simulink library "jMPClib"  (R2022b)
settings: Solver=ode45  StartTime=0.0  StopTime=10.0  RelTol=1e-3  EnableMultiTasking=on
undefined symbols (not defined in the file or in its folder): iter, lam0, MPC1, Plant, sigma, t0, titles, tlim, tol, vrw, ylims, z0
libraries: simulink x2, dspindex x2, $bdroot x1
settings Model: Creator=jocurrie  LastModifiedBy=Jonathan Currie
settings SolverCC: AlgebraicLoopSolver=TrustRegion
settings DataIOCC: LimitDataPoints=on  SaveFormat=Array  SignalLoggingSaveFormat=ModelDataLogs  ReturnWorkspaceOutputs=off
settings OptimizationCC: ExpressionDepthLimit=2147483647  LifeSpan=inf
settings DebuggingCC: UnderspecifiedInitializationDetection=Classic  MergeDetectMultiDrivingBlocksExec=none  SolverPrmCheckMsg=warning  FcnCallInpInsideContextMsg=warning  UnconnectedInputMsg=warning  UnconnectedOutputMsg=warning  UnconnectedLineMsg=warning  StateNameClashWarn=warning  SFUnexpectedBacktrackingDiag=warning  SFNoUnconditionalDefaultTransitionDiag=warning  SFExecutionAtInitializationDiag=none  SFMachineParentedDataDiag=warning  ArithmeticOperatorsInVariantConditions=warning
settings HardwareCC: ProdBitPerPointer=32  ProdBitPerSizeT=32  ProdBitPerPtrDiffT=32  ProdLargestAtomicFloat=None  ProdIntDivRoundTo=Undefined  ProdEndianess=Unspecified  ProdWordSize=32  ProdHWDeviceType=32-bit Generic
settings ModelReferenceCC: PropagateSignalLabelsOutOfModel=off
settings SFSimCC: SimUseLocalCustomCode=off  CustomCodeUndefinedFunction=UseInterfaceOnly
settings RTWCC: RTWUseLocalCustomCode=off
settings CodeAppCC: StateflowObjectComments=on
settings GRTTargetCC: TargetLangStandard=C89/C90 (ANSI)  CombineOutputUpdateFcns=off  GRTInterface=on
settings ConfigComp: CovMetricSettings=dw  CovSaveCumulativeToWorkspaceVar=on  CovSaveSingleToWorkspaceVar=on  CovExternalEMLEnable=off

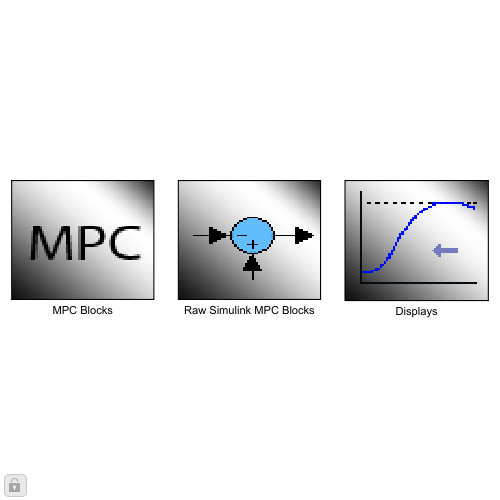
[thumbnail: Simulink's stored preview of the top-level diagram]
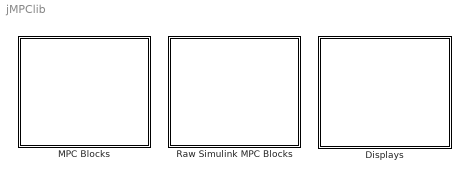
== system jMPClib ==
  Displays : Subsystem
      mask Display: image(imread('Images/scrollplot.png'))
  MPC Blocks : Subsystem
      mask Display: image(imread('Images/mpcblock.png'))
  Raw Simulink MPC Blocks : Subsystem
      mask Display: image(imread('Images/rawsim.png'))

== system jMPClib/Displays ==
  3D Simulation with Scopes : M-S-Function  FunctionName=sfun_3Dwgraph  Parameters=vrw,titles,ylims,tlim,viden  mask(jMPC 3D Simulation Interface){vrw=vrw, titles=titles, limits=ylims, tlim=tlim, viden=0}
      mask prompts: vrw "VR World"; titles "Scope Titles (Cell Array)"; limits "Scope Y Limits (Cell Array)"; tlim "Scope T Limit"; viden "Enable Video Output"
      mask help:
      | Allows the Simulink 3D interface to be run with live scrolling scopes showing runtime data.
      |
      | VR World - The VRML 3D World file name
      | Titles   - A cell array of titles to appear above each scope
      | Y Limits - A cell array of the y axis limits of each scope
      | T Limit  - The length of time before all scopes begin to scroll
      | Video Out - Enable a video output of RGB matrices. Noticeably slows down simulation!
      settings: DestroyFcn=|
      | block = get_param(gcbh, 'Parent');
      | FigHandle = get_param(block, 'UserData');
      | if ~isempty(FigHandle)
      |   close(FigHandle);
      | end
      mask Display: image(imread('Images/3Dsim.png'));
  Scrolling Display : M-S-Function  FunctionName=sfun_scroll  Parameters=Ts,Frame_Size,Update_Delay,y_lim,setp  mask(Scrolling Plot){Ts=0.1, Frame_Size=200, Update_Delay=0.005, y_lim=[-1 1], setp=on}
      mask prompts: Ts "Sampling Time (Seconds)"; Frame_Size "Frame Size (Samples)"; Update_Delay "Update Delay (Seconds)"; y_lim "Initial Y axis Limits [ymin ymax]"; setp "Enable Set Point Input"
      mask help:
      | Create a scrolling, autoscaling display for use in Simulink
      |
      | The display is a discrete component, and requires a sampling period. Adjust this period for the desired resolution.
      |
      | Frame size refers to the number of samples to be displayed on the screen before it begins to scroll.
      |
      | Note this block accepts a maximum of one input per port, if you connect a multiple dimsension signal results will be unpredictable.
      |
      | Update delay allows a rough delay of the simulation execution period, allowing the user to slow down the display.
      mask init:
      | if(~Ts)
      |     disp('Warning: Sampling Time (Ts) Not Specifed or is Zero');
      |     Ts = 0.1;
      | end
      | 
      | if(~Frame_Size)
      |     disp('Warning: Frame Size Not Specifed or is Zero');
      |     Frame_Size = 100;
      | end
      | 
      | if(Update_Delay < 0)
      |     Update_Delay = 0;
      | else if(Update_Delay > 10)
      |         disp('Warning: Update Delay Specified as > 10'); 
      |         Update_Delay = 10;
      |     end
      | end
      | 
      | if(y_lim(1) > y_lim(2))
      |     disp('Warning: Limit 1 is greater than Limit 2');
      |     y_lim(1) = -y_lim(1);
      | end
      | if(y_lim(1) == y_lim(2))
      |     disp('Warning: Limits are equal');
      |     if(~y_lim(1))
      |         y_lim(2) = 1;
      |     else
      |         y_lim(2) = y_lim(2)+abs(y_lim(2));
      |     end
      | end
      mask Help: web('jMPC_Simulink_scroll.html', '-helpbrowser');
      mask Display: image(imread('Images/Scrollpic.jpg'))

== system jMPClib/MPC Blocks ==
  Continuous ODE Plant : M-S-Function  FunctionName=sfun_jNL  Parameters=jNLObj  mask(Continuous ODE Model){jNLObj=Plant}
      mask prompts: jNLObj "jNL Object"
      mask help:
      | Implements a jNL object containing a function handle to an Ordinary Differential Equation (ODE) containing the state update equation.
      |
      | Accepts a jNL class object containing the model ODE function.
      mask Display:
      | image(imread('ode_plant.png'))
      | text(0.3,0.35,'dx/dt = f(x,u)')
      | port_label('output',1,'y ')
      | port_label('output',2,'x ')
      | port_label('input',1,' u')
  Discrete LTI Plant : Subsystem  mask(Discrete Linear Model){jSSobj=Plant}
      mask prompts: jSSobj "jSS Object"
      mask help:
      | x(k+1)  = Ax(k) + Bu(k)
      | y(k+1)  = Cx(k+1)
      |
      | Accepts a jSS class object containing the model SS matrices.
      mask Help: web('jMPC_Simulink_displant.html', '-helpbrowser');
      mask Display:
      | image(imread('Images/ltiplant.png'))
      | text(0.3,0.35,'x+1 = Ax+Bu')
      | port_label('output',1,'y ')
      | port_label('output',2,'x ')
      | port_label('input',1,' u')
  Discrete MPC Controller : Subsystem  mask(Model Predictive Controller){SIMJMPC=MPC1}
      mask prompts: SIMJMPC "jMPC Object"
      mask help:
      | MPC implemented as a C-MEX S Function for accelerated MPC simulations.
      |
      | Accepts a jMPC class object containing the controller specification.
      mask Help: web('jMPC_Simulink_dismpcs.html', '-helpbrowser');
      mask Display:
      | image(imread('Images/MPCPic.png'));
      | port_label('input',1,'mdist');
      | port_label('input',2,'setp');
      | port_label('input',3,'yp');
      | port_label('output',1,'u');
      | port_label('output',2,'delu');
      | port_label('output',4,'xm');
      | port_label('output',3,'ym');
      | port_label('output',5,'stats');

== system jMPClib/Raw Simulink MPC Blocks ==
  Discrete MPC (Raw Simulink) : Subsystem  mask(Model Predictive Controller){J=MPC1}
      mask prompts: J "jMPC Object"
      mask help:
      | General MPC for simulation (states and model output viewable).
      |
      | Accepts a jMPC class object containing the controller specification.
      mask Help: web('jMPC_Simulink_dismpc.html', '-helpbrowser');
      mask Display:
      | image(imread('Images/MPCPic2.png'));
      | port_label('input',1,'setp');
      | port_label('input',2,'yp');
      | port_label('output',1,'u');
      | port_label('output',2,'delu');
      | port_label('output',4,'xm');
      | port_label('output',3,'ym');
  Wright QP Solver : Subsystem  mask(Quadratic Programming Solver){iter=iter, tol=tol, z0=z0, lam0=lam0, t0=t0, esig=sigma}
      mask prompts: iter "Maximum Iterations"; tol "Solver Tolerance"; z0 "Initial z (ndec x 1)"; lam0 "Initial lambda (ncon x 1)"; t0 "Initial t (ncon x 1)"; esig "Sigma Array (ncon x 1)"
      mask help: QP Solver for MPC using Wright's Method
      mask Help: web('jMPC_Simulink_wright.html', '-helpbrowser');
      mask Display:
      | image(imread('Images/WrightPic.jpg'));
      | port_label('input',1,'H');
      | port_label('input',2,'f');
      | port_label('input',3,'A');
      | port_label('input',4,'b');
      | port_label('output',1,'Solution');
      | port_label('output',2,'Iterations');

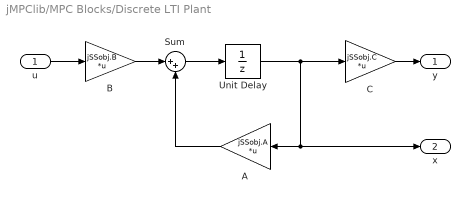
== system jMPClib/MPC Blocks/Discrete LTI Plant ==
  u : Inport
  A : Gain  Gain=jSSobj.A  Multiplication=Matrix(K*u)
  B : Gain  Gain=jSSobj.B  Multiplication=Matrix(K*u)
  C : Gain  Gain=jSSobj.C  Multiplication=Matrix(K*u)
  Sum : Sum  Inputs=|++
  Unit Delay : UnitDelay  InitialCondition=jSSobj.x0  SampleTime=-1  HasFrameUpgradeWarning=on
  y : Outport
  x : Outport  Port=2
  wires:
  C/1 -> y/1
  u/1 -> B/1
  Sum/1 -> Unit Delay/1
  B/1 -> Sum/1
  A/1 -> Sum/2
  Unit Delay/1 -> x/1, A/1, C/1

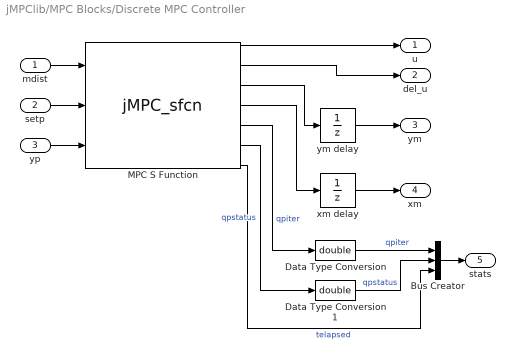
== system jMPClib/MPC Blocks/Discrete MPC Controller ==
  mdist : Inport
  setp : Inport  Port=2
  yp : Inport  Port=3
  Bus Creator : BusCreator  Inputs=3
  Data Type Conversion : DataTypeConversion  OutDataTypeStr=double  SaturateOnIntegerOverflow=off  RndMeth=Floor
  Data Type Conversion1 : DataTypeConversion  OutDataTypeStr=double  SaturateOnIntegerOverflow=off  RndMeth=Floor
  MPC S Function : S-Function  FunctionName=jMPC_sfcn  Parameters=SIMJMPC.Model.A,SIMJMPC.Model.B,SIMJMPC.Model.Ts,SIMJMPC.Np,SIMJMPC.Nb,SIMJMPC.pred,SIMJMPC.sizes,SIMJMPC.state_est,SIMJMPC.QP,SIMJMPC.index,SIMJMPC.constraints,SIMJMPC.initial,SIMJMPC.mpcopts,SIMJMPC.lin  SFunctionDeploymentMode=off  EnableBusSupport=off
  xm delay : UnitDelay  InitialCondition=SIMJMPC.initial.xm+SIMJMPC.lin.x_op  SampleTime=-1  HasFrameUpgradeWarning=on
  ym delay : UnitDelay  InitialCondition=SIMJMPC.initial.ym+SIMJMPC.lin.y_op_full  SampleTime=-1  HasFrameUpgradeWarning=on
  u : Outport
  del_u : Outport  Port=2
  ym : Outport  Port=3
  xm : Outport  Port=4
  stats : Outport  Port=5
  wires:
  MPC S Function/7 -> Bus Creator/3  "telapsed"
  Bus Creator/1 -> stats/1
  MPC S Function/3 -> ym delay/1
  MPC S Function/4 -> xm delay/1
  MPC S Function/1 -> u/1
  MPC S Function/2 -> del_u/1
  ym delay/1 -> ym/1
  xm delay/1 -> xm/1
  mdist/1 -> MPC S Function/1
  setp/1 -> MPC S Function/2
  yp/1 -> MPC S Function/3
  Data Type Conversion1/1 -> Bus Creator/2  "qpstatus"
  Data Type Conversion/1 -> Bus Creator/1  "qpiter"
  MPC S Function/5 -> Data Type Conversion/1  "qpiter"
  MPC S Function/6 -> Data Type Conversion1/1  "qpstatus"

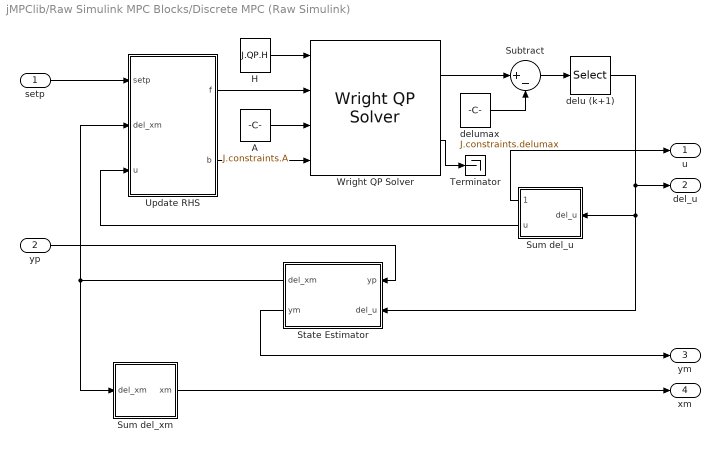
== system jMPClib/Raw Simulink MPC Blocks/Discrete MPC (Raw Simulink) ==
  setp : Inport
  yp : Inport  Port=2
  A : Constant  Value=J.constraints.A
  H : Constant  Value=J.QP.H
  State Estimator : Subsystem
  Subtract : Sum  Inputs=|+-
  Sum del_u : Subsystem
  Sum del_xm : Subsystem
  Terminator : Terminator
  Update RHS : Subsystem
  Wright QP Solver : $bdroot/Raw Simulink MPC Blocks/Wright QP Solver  iter=200  tol=1e-6  z0=J.QP.z0  lam0=J.QP.lam0  t0=J.QP.t0  esig=J.QP.sigma
  delu (k+1) : Selector  InputPortWidth=J.sizes.Nb_in  IndexOptions=Index vector (dialog)  Indices=1:J.sizes.n_in  OutputSizes=1
  delumax : Constant  Value=J.constraints.delumax
  u : Outport
  del_u : Outport  Port=2
  ym : Outport  Port=3
  xm : Outport  Port=4
  wires:
  H/1 -> Wright QP Solver/1
  A/1 -> Wright QP Solver/3
  Update RHS/1(f) -> Wright QP Solver/2
  Update RHS/2(b) -> Wright QP Solver/4
  Wright QP Solver/2 -> Terminator/1
  Wright QP Solver/1 -> Subtract/1
  Subtract/1 -> delu (k+1)/1
  delu (k+1)/1 -> del_u/1, State Estimator/2(del_u), Sum del_u/1(del_u)
  setp/1 -> Update RHS/1(setp)
  delumax/1 -> Subtract/2
  State Estimator/1(del_xm) -> Update RHS/2(del_xm), Sum del_xm/1(del_xm)
  yp/1 -> State Estimator/1(yp)
  Sum del_xm/1(xm) -> xm/1
  State Estimator/2(ym) -> ym/1
  Sum del_u/1(u (k+1)) -> u/1
  Sum del_u/2(u) -> Update RHS/3(u)

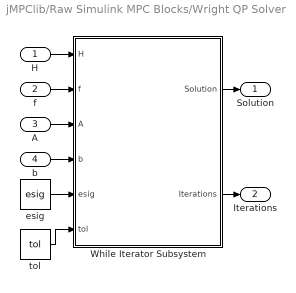
== system jMPClib/Raw Simulink MPC Blocks/Wright QP Solver ==
  H : Inport
  f : Inport  Port=2
  A : Inport  Port=3
  b : Inport  Port=4
  While Iterator Subsystem : Subsystem  TreatAsAtomicUnit=on
  esig : Constant  Value=esig
  tol : Constant  Value=tol
  Solution : Outport
  Iterations : Outport  Port=2
  wires:
  While Iterator Subsystem/2(Iterations) -> Iterations/1
  While Iterator Subsystem/1(Solution) -> Solution/1
  tol/1 -> While Iterator Subsystem/6(tol)
  esig/1 -> While Iterator Subsystem/5(esig)
  b/1 -> While Iterator Subsystem/4(b)
  A/1 -> While Iterator Subsystem/3(A)
  H/1 -> While Iterator Subsystem/1(H)
  f/1 -> While Iterator Subsystem/2(f)

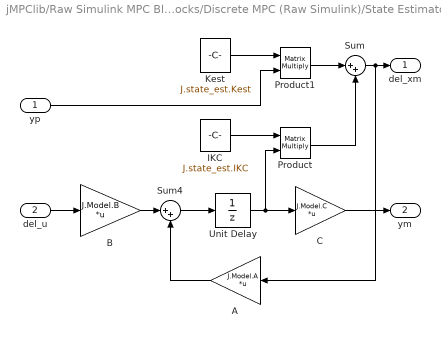
== system jMPClib/Raw Simulink MPC Blocks/Discrete MPC (Raw Simulink)/State Estimator ==
  yp : Inport
  del_u : Inport  Port=2
  A : Gain  Gain=J.Model.A  Multiplication=Matrix(K*u)
  B : Gain  Gain=J.Model.B  Multiplication=Matrix(K*u)
  C : Gain  Gain=J.Model.C  Multiplication=Matrix(K*u)
  IKC : Constant  Value=J.state_est.IKC
  Kest : Constant  Value=J.state_est.Kest
  Product : Product  Multiplication=Matrix(*)  RndMeth=Zero
  Product1 : Product  Multiplication=Matrix(*)  RndMeth=Zero
  Sum : Sum  Inputs=|++
  Sum4 : Sum  Inputs=|++
  Unit Delay : UnitDelay  InitialCondition=J.Model.x0  SampleTime=-1  HasFrameUpgradeWarning=on
  del_xm : Outport
  ym : Outport  Port=2
  wires:
  IKC/1 -> Product/1
  Kest/1 -> Product1/1
  yp/1 -> Product1/2
  Product1/1 -> Sum/1
  Product/1 -> Sum/2
  Unit Delay/1 -> Product/2, C/1
  Sum/1 -> del_xm/1, A/1
  B/1 -> Sum4/1
  Sum4/1 -> Unit Delay/1
  A/1 -> Sum4/2
  del_u/1 -> B/1
  C/1 -> ym/1

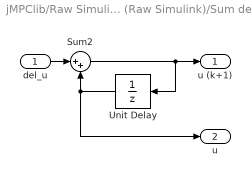
== system jMPClib/Raw Simulink MPC Blocks/Discrete MPC (Raw Simulink)/Sum del_u ==
  del_u : Inport
  Sum2 : Sum  Inputs=|++
  Unit Delay : UnitDelay  InitialCondition=J.initial.u  SampleTime=-1  HasFrameUpgradeWarning=on
  u (k+1) : Outport
  u : Outport  Port=2
  wires:
  Unit Delay/1 -> Sum2/2, u/1
  del_u/1 -> Sum2/1
  Sum2/1 -> Unit Delay/1, u (k+1)/1

== system jMPClib/Raw Simulink MPC Blocks/Discrete MPC (Raw Simulink)/Sum del_xm ==
  del_xm : Inport
  Sum1 : Sum  Inputs=|++
  Unit Delay1 : UnitDelay  InitialCondition=J.initial.xm  SampleTime=-1  HasFrameUpgradeWarning=on
  xm_select : Selector  InputPortWidth=J.sizes.states+J.sizes.n_out  IndexOptions=Index vector (dialog)  Indices=1:J.sizes.states  OutputSizes=1
  xm : Outport
  wires:
  Sum1/1 -> Unit Delay1/1, xm/1
  Unit Delay1/1 -> Sum1/2
  xm_select/1 -> Sum1/1
  del_xm/1 -> xm_select/1

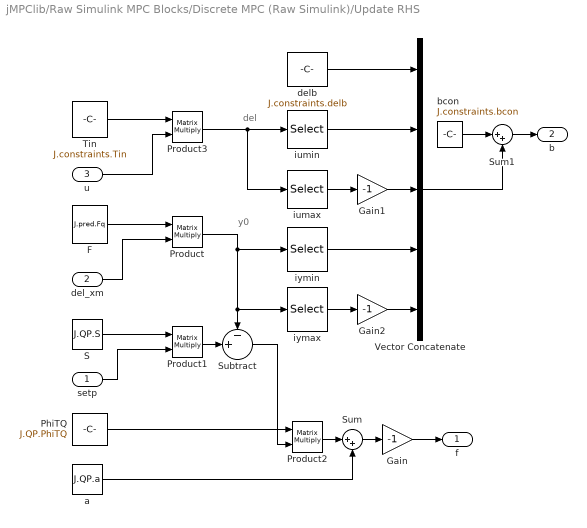
== system jMPClib/Raw Simulink MPC Blocks/Discrete MPC (Raw Simulink)/Update RHS ==
  note: del
  note: y0
  setp : Inport
  del_xm : Inport  Port=2
  u : Inport  Port=3
  F : Constant  Value=J.pred.Fq
  Gain : Gain  Gain=-1
  Gain1 : Gain  Gain=-1
  Gain2 : Gain  Gain=-1
  PhiTQ : Constant  Value=J.QP.PhiTQ
  Product{,1..3} (4 alike) : Product  Multiplication=Matrix(*)  RndMeth=Zero
  S : Constant  Value=J.QP.S
  Subtract : Sum  Inputs=-+|
  Sum : Sum  Inputs=|++
  Sum1 : Sum  Inputs=|++
  Tin : Constant  Value=J.constraints.Tin
  Vector Concatenate : Concatenate  NumInputs=5
  a : Constant  Value=J.QP.a
  bcon : Constant  Value=J.constraints.bcon
  delb : Constant  Value=J.constraints.delb
  iumax : Selector  InputPortWidth=J.sizes.Nb_in  IndexOptions=Index vector (dialog)  Indices=J.constraints.iumax  OutputSizes=1
  iumin : Selector  InputPortWidth=J.sizes.Nb_in  IndexOptions=Index vector (dialog)  Indices=J.constraints.iumin  OutputSizes=1
  iymax : Selector  InputPortWidth=J.sizes.Np_out  IndexOptions=Index vector (dialog)  Indices=J.constraints.iymax  OutputSizes=1
  iymin : Selector  InputPortWidth=J.sizes.Np_out  IndexOptions=Index vector (dialog)  Indices=J.constraints.iymin  OutputSizes=1
  f : Outport
  b : Outport  Port=2
  wires:
  Gain/1 -> f/1
  Sum1/1 -> b/1
  Vector Concatenate/1 -> Sum1/2
  bcon/1 -> Sum1/1
  Gain2/1 -> Vector Concatenate/5
  Gain1/1 -> Vector Concatenate/3
  Product3/1 -> iumin/1, iumax/1
  delb/1 -> Vector Concatenate/1
  u/1 -> Product3/2
  Tin/1 -> Product3/1
  Sum/1 -> Gain/1
  Subtract/1 -> Product2/2
  PhiTQ/1 -> Product2/1
  a/1 -> Sum/2
  Product2/1 -> Sum/1
  setp/1 -> Product1/2
  S/1 -> Product1/1
  del_xm/1 -> Product/2
  F/1 -> Product/1
  iumin/1 -> Vector Concatenate/2
  iumax/1 -> Gain1/1
  iymax/1 -> Gain2/1
  Product1/1 -> Subtract/2
  iymin/1 -> Vector Concatenate/4
  Product/1 -> iymin/1, iymax/1, Subtract/1

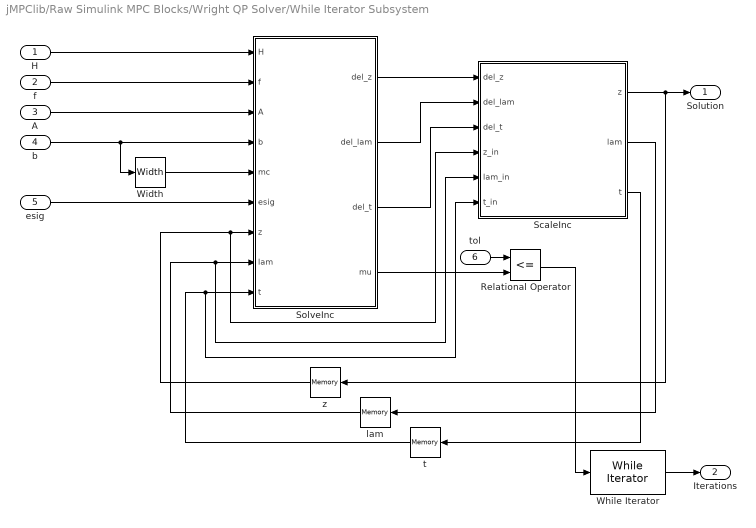
== system jMPClib/Raw Simulink MPC Blocks/Wright QP Solver/While Iterator Subsystem ==
  H : Inport
  f : Inport  Port=2
  A : Inport  Port=3
  b : Inport  Port=4
  esig : Inport  Port=5
  tol : Inport  Port=6
  Relational Operator : RelationalOperator  Operator=<=  OutDataTypeStr=boolean  InputSameDT=off
  ScaleInc : Subsystem
  SolveInc : Subsystem
  While Iterator : WhileIterator  MaxIters=iter  WhileBlockType=do-while  ResetStates=reset  ShowIterationPort=on  OutputDataType=double
  Width : Width
  lam : Memory  InitialCondition=lam0  InheritSampleTime=on
  t : Memory  InitialCondition=t0  InheritSampleTime=on
  z : Memory  InitialCondition=z0  InheritSampleTime=on
  Solution : Outport  OutDataTypeStr=double
  Iterations : Outport  Port=2  OutDataTypeStr=double
  wires:
  Width/1 -> SolveInc/5(mc)
  tol/1 -> Relational Operator/1
  SolveInc/4(mu) -> Relational Operator/2
  Relational Operator/1 -> While Iterator/1
  While Iterator/1 -> Iterations/1
  t/1 -> ScaleInc/6(t_in), SolveInc/9(t)
  lam/1 -> ScaleInc/5(lam_in), SolveInc/8(lam)
  z/1 -> ScaleInc/4(z_in), SolveInc/7(z)
  ScaleInc/3(t) -> t/1
  ScaleInc/2(lam) -> lam/1
  ScaleInc/1(z) -> z/1, Solution/1
  esig/1 -> SolveInc/6(esig)
  b/1 -> Width/1, SolveInc/4(b)
  A/1 -> SolveInc/3(A)
  f/1 -> SolveInc/2(f)
  H/1 -> SolveInc/1(H)
  SolveInc/3(del_t) -> ScaleInc/3(del_t)
  SolveInc/2(del_lam) -> ScaleInc/2(del_lam)
  SolveInc/1(del_z) -> ScaleInc/1(del_z)

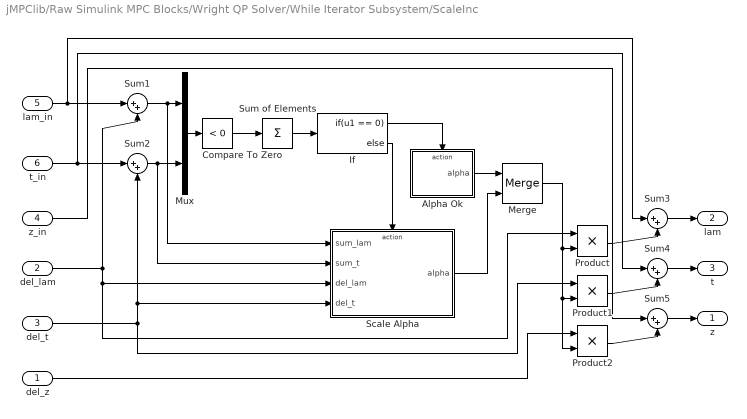
== system jMPClib/Raw Simulink MPC Blocks/Wright QP Solver/While Iterator Subsystem/ScaleInc ==
  del_z : Inport
  del_lam : Inport  Port=2
  del_t : Inport  Port=3
  z_in : Inport  Port=4
  lam_in : Inport  Port=5
  t_in : Inport  Port=6
  Alpha Ok : Subsystem  TreatAsAtomicUnit=on
  Compare To Zero : simulink/Logic and Bit Operations/Compare To Zero  relop=<  OutDataTypeStr=boolean  ZeroCross=off
  If : If  IfExpression=u1 == 0
  Merge : Merge
  Mux : Mux  Inputs=2
  Product : Product  RndMeth=Zero
  Product1 : Product  RndMeth=Zero
  Product2 : Product  RndMeth=Zero
  Scale Alpha : Subsystem  TreatAsAtomicUnit=on
  Sum of Elements : Sum  Inputs=+
  Sum{1..5} (5 alike) : Sum  Inputs=|++
  z : Outport
  lam : Outport  Port=2
  t : Outport  Port=3
  wires:
  Sum2/1 -> Mux/2, Scale Alpha/2(sum_t)
  Mux/1 -> Compare To Zero/1
  Compare To Zero/1 -> Sum of Elements/1
  Sum1/1 -> Mux/1, Scale Alpha/1(sum_lam)
  Sum of Elements/1 -> If/1
  If/1 -> Alpha Ok/Action
  Alpha Ok/1(alpha) -> Merge/1
  Scale Alpha/1(alpha) -> Merge/2
  lam_in/1 -> Sum1/1, Sum3/1
  t_in/1 -> Sum2/1, Sum4/1
  del_lam/1 -> Sum1/2, Product/1, Scale Alpha/3(del_lam)
  del_t/1 -> Product1/1, Sum2/2, Scale Alpha/4(del_t)
  If/2 -> Scale Alpha/Action
  Merge/1 -> Product/2, Product1/2, Product2/2
  Product/1 -> Sum3/2
  Product1/1 -> Sum4/2
  Product2/1 -> Sum5/2
  z_in/1 -> Sum5/1
  del_z/1 -> Product2/1
  Sum3/1 -> lam/1
  Sum4/1 -> t/1
  Sum5/1 -> z/1

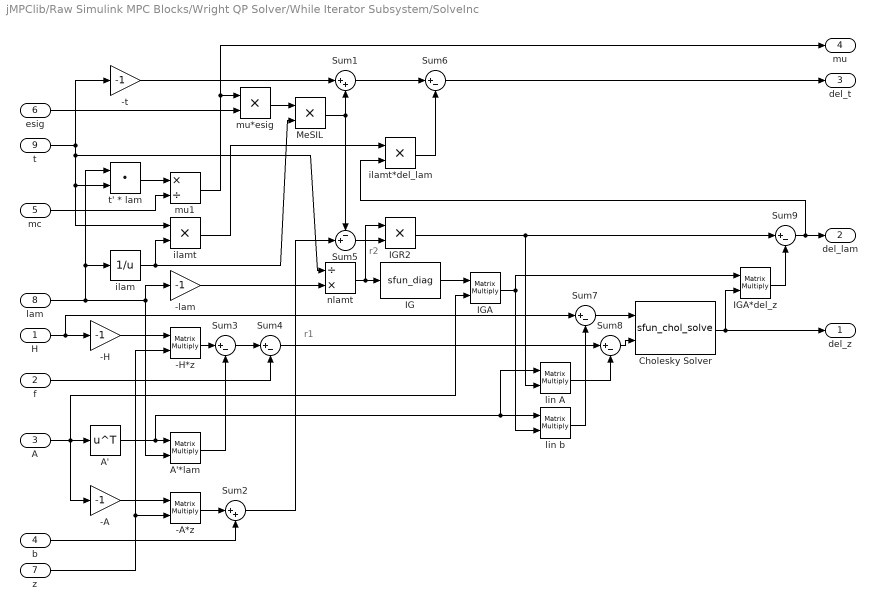
== system jMPClib/Raw Simulink MPC Blocks/Wright QP Solver/While Iterator Subsystem/SolveInc ==
  note: r1
  note: r2
  H : Inport
  f : Inport  Port=2
  A : Inport  Port=3
  b : Inport  Port=4
  mc : Inport  Port=5
  esig : Inport  Port=6
  z : Inport  Port=7
  lam : Inport  Port=8
  t : Inport  Port=9
  -A : Gain  Gain=-1
  -A*z : Product  Multiplication=Matrix(*)  RndMeth=Zero
  -H : Gain  Gain=-1
  -H*z : Product  Multiplication=Matrix(*)  RndMeth=Zero
  -lam : Gain  Gain=-1
  -t : Gain  Gain=-1
  A' : Math  Operator=transpose  SignedPower=on
  A'*lam : Product  Multiplication=Matrix(*)  RndMeth=Zero
  Cholesky Solver : M-S-Function  FunctionName=sfun_chol_solve  Parameters=err  mask(Cholesky Solver){err=Warning}
      mask prompts: err "Not Positive Definite Action"
      mask help: Solve Hx = f using a Cholesky Factorization. H must be a square symmetrix positive definite matrix. f must have the same number of rows as H.
      mask TypeOptions err: Ignore | Warning | Error
      mask Display:
      | text(0.20,0.6,'R = chol(H)');
      | text(0.22,0.4,'x = R\(R''\f)');
      | port_label('input',1,'H')
      | port_label('input',2,'f')
      | port_label('output',1,'x')
  IG : M-S-Function  FunctionName=sfun_diag  mask(Diagonalize){}
      mask help: Convert a vector of elements to the diagonal in a full matrix.
      mask Display:
      | text(0.30,0.5,'D =\ndiag(D)');
      | port_label('input',1,'d')
      | port_label('output',1,'D')
  IGA : Product  Multiplication=Matrix(*)  RndMeth=Zero
  IGA*del_z : Product  Multiplication=Matrix(*)  RndMeth=Zero
  IGR2 : Product  RndMeth=Zero
  MeSIL : Product  RndMeth=Zero
  Sum1 : Sum  Inputs=|++
  Sum2 : Sum  Inputs=|++
  Sum{3..4,6..9} (6 alike) : Sum  Inputs=|+-
  Sum5 : Sum  Inputs=-+|
  ilam : Math  Operator=reciprocal  SignedPower=on
  ilamt : Product  RndMeth=Zero
  ilamt*del_lam : Product  RndMeth=Zero
  lin A : Product  Multiplication=Matrix(*)  RndMeth=Zero
  lin b : Product  Multiplication=Matrix(*)  RndMeth=Zero
  mu*esig : Product  RndMeth=Zero
  mu1 : Product  Inputs=*/
  nlamt : Product  Inputs=/*
  t' * lam : DotProduct  OutDataTypeStr=Inherit: Inherit via internal rule
  del_z : Outport
  del_lam : Outport  Port=2
  del_t : Outport  Port=3
  mu : Outport  Port=4
  wires:
  z/1 -> -H*z/2, -A*z/2
  b/1 -> Sum2/2
  f/1 -> Sum4/2
  H/1 -> -H/1, Sum7/1
  mc/1 -> mu1/2
  esig/1 -> mu*esig/2
  Sum6/1 -> del_t/1
  ilamt*del_lam/1 -> Sum6/2
  Sum1/1 -> Sum6/1
  -t/1 -> Sum1/1
  IGA*del_z/1 -> Sum9/2
  Cholesky Solver/1 -> del_z/1, IGA*del_z/2
  Sum8/1 -> Cholesky Solver/2
  lin A/1 -> Sum8/2
  IGR2/1 -> lin A/2, Sum9/1
  Sum7/1 -> Cholesky Solver/1
  lin b/1 -> Sum7/2
  Sum5/1 -> IGR2/2
  -A*z/1 -> Sum2/1
  -A/1 -> -A*z/1
  Sum4/1 -> Sum8/1
  A'*lam/1 -> Sum3/2
  -H*z/1 -> Sum3/1
  A'/1 -> lin A/1, lin b/1, A'*lam/1
  A/1 -> A'/1, -A/1, IGA/2
  -H/1 -> -H*z/1
  ilam/1 -> MeSIL/2, ilamt/2
  MeSIL/1 -> Sum5/1, Sum1/2
  mu*esig/1 -> MeSIL/1
  mu1/1 -> mu*esig/1, mu/1
  t' * lam/1 -> mu1/1
  lam/1 -> t' * lam/1, ilam/1, A'*lam/2, -lam/1
  Sum3/1 -> Sum4/1
  ilamt/1 -> ilamt*del_lam/1
  Sum2/1 -> Sum5/2
  IG/1 -> IGA/1
  t/1 -> -t/1, ilamt/1, t' * lam/2, nlamt/1
  nlamt/1 -> IGR2/1, IG/1
  -lam/1 -> nlamt/2
  IGA/1 -> lin b/2, IGA*del_z/1
  Sum9/1 -> ilamt*del_lam/2, del_lam/1

== system jMPClib/Raw Simulink MPC Blocks/Wright QP Solver/While Iterator Subsystem/ScaleInc/Alpha Ok ==
  Action Port : ActionPort  PropagateVarSize=During execution
  Constant : Constant
  alpha : Outport  InitialOutput=1
  wires:
  Constant/1 -> alpha/1

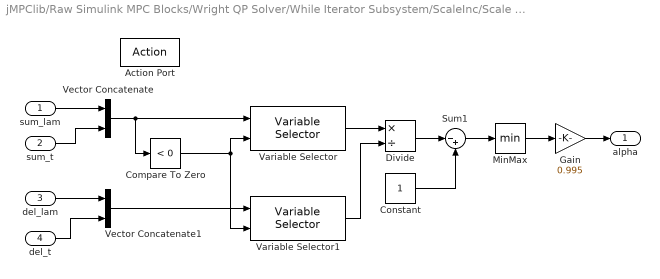
== system jMPClib/Raw Simulink MPC Blocks/Wright QP Solver/While Iterator Subsystem/ScaleInc/Scale Alpha ==
  sum_lam : Inport
  sum_t : Inport  Port=2
  del_lam : Inport  Port=3
  del_t : Inport  Port=4
  Action Port : ActionPort  PropagateVarSize=During execution
  Compare To Zero : simulink/Logic and Bit Operations/Compare To Zero  relop=<  OutDataTypeStr=boolean  ZeroCross=off
  Constant : Constant
  Divide : Product  Inputs=*/
  Gain : Gain  Gain=0.995
  MinMax : MinMax
  Sum1 : Sum  Inputs=|-+
  Variable Selector : dspindex/Variable Selector  NumInputs=1  rowsOrCols=Rows  IdxMode=Variable  Elements=[1 3]  ZerOneIdxMode=One-based  errmode=Clip Index  FillMode=on  FillValues=0
  Variable Selector1 : dspindex/Variable Selector  NumInputs=1  rowsOrCols=Rows  IdxMode=Variable  Elements=[1 3]  ZerOneIdxMode=One-based  errmode=Clip Index  FillMode=on  FillValues=1
  Vector Concatenate : Concatenate
  Vector Concatenate1 : Concatenate
  alpha : Outport
  wires:
  sum_lam/1 -> Vector Concatenate/1
  sum_t/1 -> Vector Concatenate/2
  del_lam/1 -> Vector Concatenate1/1
  del_t/1 -> Vector Concatenate1/2
  Divide/1 -> Sum1/1
  Sum1/1 -> MinMax/1
  MinMax/1 -> Gain/1
  Gain/1 -> alpha/1
  Vector Concatenate/1 -> Compare To Zero/1, Variable Selector/1
  Vector Concatenate1/1 -> Variable Selector1/1
  Compare To Zero/1 -> Variable Selector1/2, Variable Selector/2
  Variable Selector1/1 -> Divide/2
  Variable Selector/1 -> Divide/1
  Constant/1 -> Sum1/2
